simulink model "DCM"  (R2021b)
settings: Solver=VariableStepAuto  StartTime=0.0  StopTime=10.0  RelTol=1e-3
values from neighbouring files (symbols this model uses):
  A0 = eye(3)    [Lab08_script.m]    (also in Lab7_script.m; Lab7_scriptscalar.m; Lab_GG.m)
  J = [Ixx 0 0; 0 Iyy 0; 0 0 Izz]    [euler_equation_tasks.m]    (also in lab5_task2.m)
  Jinv = inv(J)    [euler_equation_tasks.m]    (also in lab5_task2.m)
  w0 = [0.45 0.52 0.55]'    [euler_equation_tasks.m]    (also in lab5_task2.m = [C 0.1 0.1]')
libraries: matrix_library x1
settings Model: Creator=arilu  LastModifiedBy=arilu

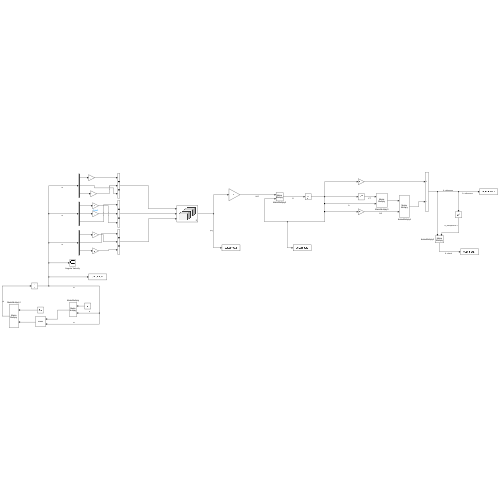
[thumbnail: Simulink's stored preview of the top-level diagram]
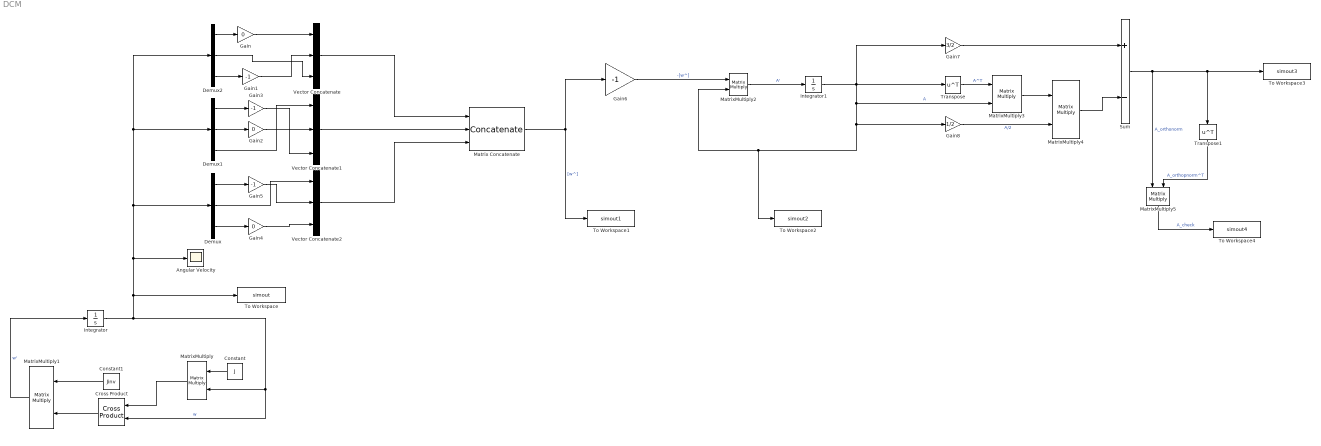
== system DCM ==
  Angular Velocity : Scope
  Constant : Constant  Value=J
  Constant1 : Constant  Value=Jinv
  Cross Product : matrix_library/Cross Product
      settings: SourceProductBaseCode=SL
  Demux : Demux  Outputs=3
  Demux1 : Demux  Outputs=3
  Demux2 : Demux  Outputs=3
  Gain : Gain  Gain=0
  Gain{1,3,5..6} (4 alike) : Gain  Gain=-1
  Gain2 : Gain  Gain=0
  Gain4 : Gain  Gain=0
  Gain7 : Gain  Gain=3/2
  Gain8 : Gain  Gain=1/2
  Integrator : Integrator  InitialCondition=w0
  Integrator1 : Integrator  InitialCondition=A0
  Matrix Concatenate : Concatenate  NumInputs=3  Mode=Multidimensional array  ConcatenateDimension=2
  MatrixMultiply{,1..5} (6 alike) : Product  Multiplication=Matrix(*)
  Sum : Sum  Inputs=+-
  To Workspace : ToWorkspace  VariableName=simout  SampleTime=-1
  To Workspace1 : ToWorkspace  VariableName=simout1  SampleTime=-1
  To Workspace2 : ToWorkspace  VariableName=simout2  SampleTime=-1
  To Workspace3 : ToWorkspace  VariableName=simout3  SampleTime=-1
  To Workspace4 : ToWorkspace  VariableName=simout4  SampleTime=-1
  Transpose : Math  Operator=transpose  SaturateOnIntegerOverflow=on
  Transpose1 : Math  Operator=transpose  SaturateOnIntegerOverflow=on
  Vector Concatenate : Concatenate  NumInputs=3
  Vector Concatenate1 : Concatenate  NumInputs=3
  Vector Concatenate2 : Concatenate  NumInputs=3
  wires:
  MatrixMultiply/1 -> Cross Product/1
  Integrator/1 -> To Workspace/1, Demux1/1, Demux2/1, Demux/1, Angular Velocity/1, Cross Product/2, MatrixMultiply/2  "w"
  MatrixMultiply1/1 -> Integrator/1  "w'"
  Constant/1 -> MatrixMultiply/1
  Cross Product/1 -> MatrixMultiply1/2
  Constant1/1 -> MatrixMultiply1/1
  Demux2/1 -> Gain/1
  Gain/1 -> Vector Concatenate/1
  Demux2/3 -> Gain1/1
  Demux1/2 -> Gain2/1
  Gain2/1 -> Vector Concatenate1/2
  Demux1/1 -> Gain3/1
  Demux/3 -> Gain4/1
  Demux/1 -> Gain5/1
  Gain4/1 -> Vector Concatenate2/3
  Vector Concatenate/1 -> Matrix Concatenate/1
  Vector Concatenate1/1 -> Matrix Concatenate/2
  Vector Concatenate2/1 -> Matrix Concatenate/3
  Matrix Concatenate/1 -> To Workspace1/1, Gain6/1  "[w^]"
  MatrixMultiply2/1 -> Integrator1/1  "A'"
  Integrator1/1 -> To Workspace2/1, MatrixMultiply2/2, Gain8/1, MatrixMultiply3/2, Transpose/1, Gain7/1  "A"
  Gain6/1 -> MatrixMultiply2/1  "-[w^]"
  Transpose/1 -> MatrixMultiply3/1  "A^T"
  Gain7/1 -> Sum/1
  Gain8/1 -> MatrixMultiply4/2  "A/2"
  MatrixMultiply3/1 -> MatrixMultiply4/1
  MatrixMultiply4/1 -> Sum/2
  Sum/1 -> Transpose1/1, To Workspace3/1, MatrixMultiply5/1  "A_orthonorm"
  Transpose1/1 -> MatrixMultiply5/2  "A_orthopnorm^T"
  MatrixMultiply5/1 -> To Workspace4/1  "A_check"
  Gain1/1 -> Vector Concatenate/2
  Demux2/2 -> Vector Concatenate/3
  Gain3/1 -> Vector Concatenate1/3
  Demux1/3 -> Vector Concatenate1/1
  Gain5/1 -> Vector Concatenate2/2
  Demux/2 -> Vector Concatenate2/1
